simulink model "vehicleModelMatlab"  (R2021a)
settings: Solver=VariableStepAuto  StartTime=0.0  StopTime=10.0  RelTol=1e-3
values from neighbouring files (symbols this model uses):
  Iz = 1536.70    (= 1536.7)    [LaneFollowingVehicleModel.m]    (also in jacFunc.m; mainn.m; modelKating.m; modelOutputKating.m)
  lf = 1.22    [LaneFollowingVehicleModel.m]    (also in jacFunc.m; mainn.m; modelKating.m; modelOutputKating.m)
  lr = 1.36    [LaneFollowingVehicleModel.m]    (also in jacFunc.m; mainn.m; modelKating.m; modelOutputKating.m)
  m = 1500 + 2*80 + 300    (= 1960)    [LaneFollowingVehicleModel.m]    (also in jacFunc.m; mainn.m; modelKating.m; modelOutputKating.m)
undefined symbols (not defined in the file or in its folder): Cf, Cr, tau, v0
settings Model: Creator=septi  LastModifiedBy=septi

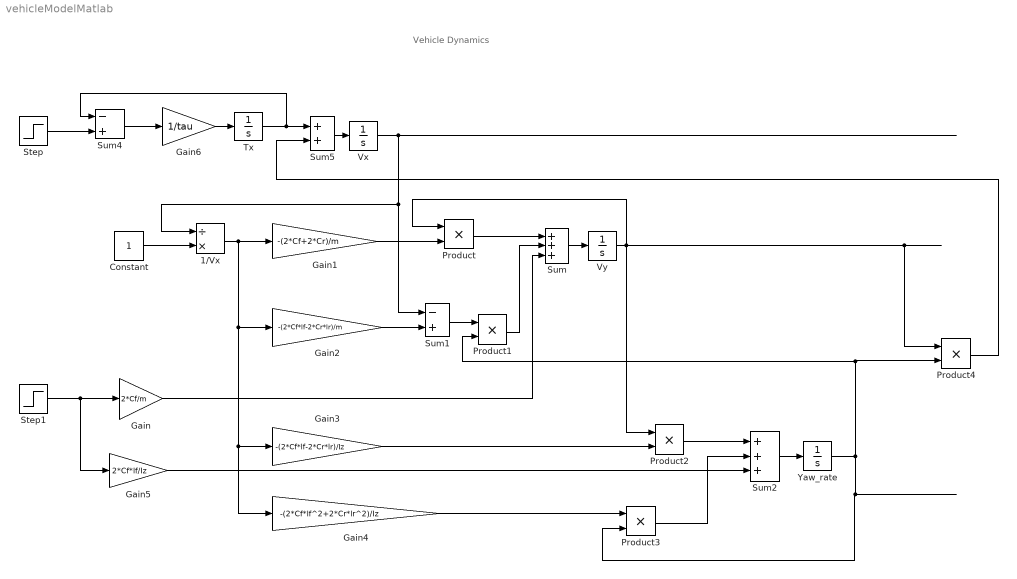
== system vehicleModelMatlab ==
  note: Vehicle Dynamics
  1/Vx : Product  Inputs=/*
  Constant : Constant
  Gain : Gain  Gain=2*Cf/m
  Gain1 : Gain  Gain=-(2*Cf+2*Cr)/m
  Gain2 : Gain  Gain=-(2*Cf*lf-2*Cr*lr)/m
  Gain3 : Gain  Gain=-(2*Cf*lf-2*Cr*lr)/Iz
  Gain4 : Gain  Gain=-(2*Cf*lf^2+2*Cr*lr^2)/Iz
  Gain5 : Gain  Gain=2*Cf*lf/Iz
  Gain6 : Gain  Gain=1/tau
  Product{,1..4} (5 alike) : Product
  Step : Step  SampleTime=0
  Step1 : Step  SampleTime=0
  Sum : Sum  Inputs=+++
  Sum1 : Sum  Inputs=-+
  Sum2 : Sum  Inputs=+++
  Sum4 : Sum  Inputs=-+
  Sum5 : Sum
  Tx : Integrator
  Vx : Integrator  InitialCondition=v0
  Vy : Integrator
  "Yaw_rate " : Integrator
  wires:
  Product1/1 -> Sum/2
  "Yaw_rate "/1 -> Product3/2, Product4/2, Product1/2
  Sum1/1 -> Product1/1
  Vy/1 -> Product/1, Product4/1, Product2/1
  Sum/1 -> Vy/1
  Step1/1 -> Gain/1, Gain5/1
  Product/1 -> Sum/1
  Gain1/1 -> Product/2
  Gain2/1 -> Sum1/2
  Tx/1 -> Sum5/1, Sum4/1
  Product4/1 -> Sum5/2
  Step/1 -> Sum4/2
  Product3/1 -> Sum2/2
  Product2/1 -> Sum2/1
  Gain/1 -> Sum/3
  Gain5/1 -> Sum2/3
  1/Vx/1 -> Gain4/1, Gain3/1, Gain2/1, Gain1/1
  Gain6/1 -> Tx/1
  Sum2/1 -> "Yaw_rate "/1
  Sum4/1 -> Gain6/1
  Constant/1 -> 1/Vx/2
  Gain4/1 -> Product3/1
  Vx/1 -> 1/Vx/1, Sum1/1
  Sum5/1 -> Vx/1
  Gain3/1 -> Product2/2
